simulink model "SAR_Quad_SITL_3D_v3"  (R2025b)
settings: Solver=ode4  StartTime=0.0  StopTime=inf  FixedStep=1/60  RelTol=1e-3
libraries: dspnetwork x5, sim3dlib x1, uavsim3dlib x1
(part 2 of 2)

== matlab function SAR_Quad_SITL_3D_v3/Edge_Command_Decoder ==
  data: raw_bytes input; target_pos_ned output size=3; gps_sensor_valid input; sim_time input; cur_pos input; cur_vel input; cur_eul input; cur_ang_vel input; min_lidar_range input; triage_code input; mission_phase output size=1; gps_valid_out output size=1; edge_ok output size=1; alt_nav_conf output size=1; yaw_cmd_deg output size=1; decoder_state output size=1; target_vel_ned output size=3; active_wp output size=1; planned_route_pts output size=[32 3]; num_route_pts output size=1
function [target_pos_ned, mission_phase, gps_valid_out, edge_ok, alt_nav_conf, yaw_cmd_deg, decoder_state, target_vel_ned, active_wp, planned_route_pts, num_route_pts] = Edge_Command_Decoder(raw_bytes, gps_sensor_valid, sim_time, cur_pos, cur_vel, cur_eul, cur_ang_vel, min_lidar_range, triage_code)
target_pos_ned = zeros(3, 1);
target_vel_ned = zeros(3, 1);
mission_phase  = 0.0;
gps_valid_out  = gps_sensor_valid;
edge_ok        = 1.0;
alt_nav_conf   = 0.95;
yaw_cmd_deg    = 0.0;
decoder_state  = 0.0;
active_wp      = 0.0;
planned_route_pts = zeros(32, 3);
num_route_pts  = 1.0;

persistent mode tgt_final user_yaw home_pos last_cmd_bytes is_init
persistent sp_pos sp_vel nav_phase
persistent corridor_wps num_corridor_wps corridor_idx smooth_yaw last_flight_yaw wp_stuck_timer
if isempty(is_init)
    is_init = true;
    mode = 0.0;
    tgt_final = [cur_pos(1); cur_pos(2); 0.0];
    user_yaw = cur_eul(3) * 180.0 / pi;
    smooth_yaw = cur_eul(3) * 180.0 / pi;
    last_flight_yaw = cur_eul(3) * 180.0 / pi;
    home_pos = [0.0; 0.0; -16.0];
    last_cmd_bytes = zeros(18, 1, 'uint8');
    sp_pos = [cur_pos(1); cur_pos(2); cur_pos(3)];
    sp_vel = [0.0; 0.0; 0.0];
    nav_phase = 0.0;
    corridor_wps = zeros(32, 3);
    corridor_wps(1, :) = [cur_pos(1), cur_pos(2), cur_pos(3)];
    num_corridor_wps = 1.0;
    corridor_idx = 1.0;
    wp_stuck_timer = 0.0;
end

% REALISTIC US CITY BLOCK GEOMETRY (Park quadrant [X: 115..190, Y: 10..90] open)
buildings = [
    -12.5,  46.0,   8.0,  80.0, -35.0, 0.0;   % Northwest Block 1
     54.0, 111.0,   8.0,  80.0, -35.0, 0.0;   % Northwest Block 2 (Red brick building)
    -12.5,  46.0, -80.0,  -8.0, -35.0, 0.0;   % Southwest Block 1
     54.0, 111.0, -80.0,  -8.0, -35.0, 0.0;   % Southwest Block 2
    195.0, 255.0,   8.0,  80.0, -35.0, 0.0;   % Far East Block (Perimeter boundary)
    129.0, 200.0, -80.0,  -8.0, -35.0, 0.0;   % Southeast Block
    -80.0, -29.0,   8.0,  80.0, -35.0, 0.0;   % West-North Block
    -80.0, -29.0, -80.0,  -8.0, -35.0, 0.0    % West-South Block
];

is_new = false;
if numel(raw_bytes) >= 18 && raw_bytes(1) == uint8(170)
    for k = 1:18
        if raw_bytes(k) ~= last_cmd_bytes(k)
            is_new = true; break;
        end
    end
else
    last_cmd_bytes = zeros(18, 1, 'uint8');
end

if is_new
    for k = 1:18; last_cmd_bytes(k) = raw_bytes(k); end
    cmd_id = double(raw_bytes(2));
    b1 = zeros(4, 1, 'uint8'); b2 = zeros(4, 1, 'uint8');
    b3 = zeros(4, 1, 'uint8'); b4 = zeros(4, 1, 'uint8');
    for bi = 1:4
        b1(bi) = raw_bytes(2 + bi); b2(bi) = raw_bytes(6 + bi);
        b3(bi) = raw_bytes(10 + bi); b4(bi) = raw_bytes(14 + bi);
    end
    p1 = double(typecast(b1, 'single'));
    p2 = double(typecast(b2, 'single'));
    p3 = double(typecast(b3, 'single'));
    p4 = double(typecast(b4, 'single'));

    plan_needed = false;
    search_needed = false;

    if cmd_id == 1.0 % TAKEOFF
        mode = 1.0;
        alt_target = max(2.5, abs(p3));
        tgt_final = [cur_pos(1); cur_pos(2); -alt_target];
        user_yaw = cur_eul(3) * 180.0 / pi;
        smooth_yaw = user_yaw;
        last_flight_yaw = user_yaw;
        nav_phase = 2.0;
        corridor_wps(1, :) = tgt_final';
        num_corridor_wps = 1.0;
        corridor_idx = 1.0;
    elseif cmd_id == 2.0 % HOLD
        mode = 2.0;
        tgt_final = [cur_pos(1); cur_pos(2); cur_pos(3)];
        user_yaw = cur_eul(3) * 180.0 / pi;
        nav_phase = 2.0;
    elseif cmd_id == 3.0 % GOTO
        mode = 3.0;
        tgt_final = [p1; p2; -abs(p3)];
        user_yaw = p4;
        plan_needed = true;
    elseif cmd_id == 4.0 % SEARCH
        mode = 4.0;
        tgt_final = [p1; p2; -abs(p3)];
        user_yaw = 0.0;
        search_needed = true;
    elseif cmd_id == 5.0 % RTL
        mode = 5.0;
        tgt_final = [home_pos(1); home_pos(2); home_pos(3)];
        user_yaw = 0.0;
        plan_needed = true;
    elseif cmd_id == 6.0 % LAND
        mode = 6.0;
        tgt_final = [cur_pos(1); cur_pos(2); 0.0];
        nav_phase = 2.0;
        corridor_wps(1, :) = tgt_final';
        num_corridor_wps = 1.0;
        corridor_idx = 1.0;
    end

    if search_needed
        z_search = tgt_final(3);
        cx = tgt_final(1); cy = tgt_final(2);
        corridor_wps = zeros(32, 3);
        corridor_wps(1, :) = [cur_pos(1), cur_pos(2), z_search];
        
        pat_type = p4;
        if pat_type >= 1.5
            % Creeping line sweep across the open park
            S = 12.0; L = 48.0;
            raw_wps = [
                cx - L/2, cy - S*2, z_search;
                cx + L/2, cy - S*2, z_search;
                cx + L/2, cy - S,   z_search;
                cx - L/2, cy - S,   z_search;
                cx - L/2, cy,       z_search;
                cx + L/2, cy,       z_search;
                cx + L/2, cy + S,   z_search;
                cx - L/2, cy + S,   z_search;
                cx - L/2, cy + S*2, z_search;
                cx + L/2, cy + S*2, z_search
            ];
        else
            S = 10.0;
            raw_wps = [
                cx,     cy,     z_search;
                cx + S, cy,     z_search;
                cx + S, cy + S, z_search;
                cx - S, cy + S, z_search;
                cx - S, cy - S, z_search;
                cx + 2*S, cy - S, z_search;
                cx + 2*S, cy + 2*S, z_search;
                cx - 2*S, cy + 2*S, z_search;
                cx - 2*S, cy - 2*S, z_search;
                cx + 3*S, cy - 2*S, z_search;
                cx + 3*S, cy + 3*S, z_search;
                cx - 3*S, cy + 3*S, z_search
            ];
        end
        
        nW = size(raw_wps, 1);
        SAFETY_MARGIN = 4.0;
        for wi = 1:nW
            wx = raw_wps(wi, 1); wy = raw_wps(wi, 2); wz = raw_wps(wi, 3);
            if wz > -34.0
                for bi = 1:size(buildings, 1)
                    bx1 = buildings(bi, 1) - SAFETY_MARGIN; bx2 = buildings(bi, 2) + SAFETY_MARGIN;
                    by1 = buildings(bi, 3) - SAFETY_MARGIN; by2 = buildings(bi, 4) + SAFETY_MARGIN;
                    if wx >= bx1 && wx <= bx2 && wy >= by1 && wy <= by2
                        d_faces = [abs(wx - bx1), abs(wx - bx2), abs(wy - by1), abs(wy - by2)];
                        [~, min_f] = min(d_faces);
                        if min_f == 1;     wx = bx1;
                        elseif min_f == 2; wx = bx2;
                        elseif min_f == 3; wy = by1;
                        else;              wy = by2;
                        end
                    end
                end
            end
            corridor_wps(wi + 1, :) = [wx, wy, wz];
        end
        num_corridor_wps = double(nW + 1);
        corridor_idx = 1.0;
        nav_phase = 1.0;
        wp_stuck_timer = 0.0;
    end

    if plan_needed
        z_target = tgt_final(3);
        c_x = cur_pos(1); c_y = cur_pos(2); c_z = cur_pos(3);
        t_x = tgt_final(1); t_y = tgt_final(2);
        
        direct_clear = false;
        if (z_target <= -34.0 && c_z <= -34.0)
            direct_clear = true;
        elseif (abs(c_y) <= 7.0 && abs(t_y) <= 7.0)
            direct_clear = true;
        elseif (abs(c_x - 120.0) <= 7.0 && abs(t_x - 120.0) <= 7.0)
            direct_clear = true;
        elseif (abs(c_x - 50.0) <= 3.5 && abs(t_x - 50.0) <= 3.5)
            direct_clear = true;
        elseif (abs(c_x + 20.0) <= 7.0 && abs(t_x + 20.0) <= 7.0)
            direct_clear = true;
        end
        
        if direct_clear
            corridor_wps = zeros(32, 3);
            corridor_wps(1, :) = [c_x, c_y, z_target];
            corridor_wps(2, :) = [t_x, t_y, z_target];
            num_corridor_wps = 2.0;
        else
            corr_axes = [-20.0, 50.0, 120.0];
            [~, idx_c] = min(abs(corr_axes - c_x));
            [~, idx_t] = min(abs(corr_axes - t_x));
            x_start_corr = corr_axes(idx_c);
            x_end_corr   = corr_axes(idx_t);
            
            corridor_wps = zeros(32, 3);
            corridor_wps(1, :) = [c_x, c_y, z_target];
            w_count = 1;
            if abs(c_y) > 6.0
                w_count = w_count + 1;
                corridor_wps(w_count, :) = [x_start_corr, c_y, z_target];
                w_count = w_count + 1;
                corridor_wps(w_count, :) = [x_start_corr, 0.0, z_target];
            else
                w_count = w_count + 1;
                corridor_wps(w_count, :) = [c_x, 0.0, z_target];
            end
            if abs(x_start_corr - x_end_corr) > 1.0
                w_count = w_count + 1;
                corridor_wps(w_count, :) = [x_end_corr, 0.0, z_target];
            end
            if abs(t_y) > 6.0
                w_count = w_count + 1;
                corridor_wps(w_count, :) = [x_end_corr, t_y, z_target];
            end
            w_count = w_count + 1;
            corridor_wps(w_count, :) = [t_x, t_y, z_target];
            num_corridor_wps = double(w_count);
        end
        corridor_idx = 1.0;
        nav_phase = 1.0;
        wp_stuck_timer = 0.0;
    end
end

if mode < 0.5
    target_pos_ned = [cur_pos(1); cur_pos(2); cur_pos(3)];
    target_vel_ned = [0.0; 0.0; 0.0];
    sp_pos = [cur_pos(1); cur_pos(2); cur_pos(3)];
    sp_vel = [0.0; 0.0; 0.0];
    yaw_cmd_deg = user_yaw;
    mission_phase = 0.0;
    active_wp = 0.0;
    decoder_state = 0.0;
    planned_route_pts = corridor_wps;
    num_route_pts = num_corridor_wps;
    return;
end

c_idx = int32(corridor_idx);
if c_idx < 1; c_idx = int32(1); end
if c_idx > int32(num_corridor_wps); c_idx = int32(num_corridor_wps); end
active_target_pos = corridor_wps(c_idx, :)';

dist_wp_actual = norm(active_target_pos(1:2) - cur_pos(1:2));
dist_wp_sp     = norm(active_target_pos(1:2) - sp_pos(1:2));
cur_speed_xy   = norm(cur_vel(1:2));
dt = 1/60;

% UNREACHABLE WAYPOINT TIMEOUT: Advance if progress stalls near a wall
if c_idx < int32(num_corridor_wps)
    if dist_wp_actual > 2.0 && min_lidar_range < 3.5 && cur_speed_xy < 0.50
        wp_stuck_timer = wp_stuck_timer + dt;
    else
        wp_stuck_timer = max(0.0, wp_stuck_timer - 0.5 * dt);
    end
    if wp_stuck_timer > 0.90
        c_idx = c_idx + 1;
        corridor_idx = double(c_idx);
        active_target_pos = corridor_wps(c_idx, :)';
        wp_stuck_timer = 0.0;
    end
end

corner_angle_deg = 0.0;
if c_idx < int32(num_corridor_wps)
    next_wp = corridor_wps(c_idx + 1, :)';
    v_in = active_target_pos(1:2) - sp_pos(1:2);
    v_out = next_wp(1:2) - active_target_pos(1:2);
    if norm(v_in) > 0.1 && norm(v_out) > 0.1
        cos_ang = dot(v_in, v_out) / (norm(v_in) * norm(v_out));
        cos_ang = max(-1.0, min(1.0, cos_ang));
        corner_angle_deg = acos(cos_ang) * 180.0 / pi;
    end
end

r_switch = max(2.0, min(4.2, 0.28 * cur_speed_xy));
if c_idx < int32(num_corridor_wps)
    if (dist_wp_actual < r_switch && dist_wp_sp < r_switch * 1.2)
        c_idx = c_idx + 1;
        corridor_idx = double(c_idx);
        active_target_pos = corridor_wps(c_idx, :)';
        wp_stuck_timer = 0.0;
    end
end

speed_xy = norm(sp_vel(1:2));
if abs(user_yaw) > 1e-3
    desired_yaw = user_yaw;
    last_flight_yaw = user_yaw;
elseif speed_xy > 0.50
    desired_yaw = atan2(sp_vel(2), sp_vel(1)) * 180.0 / pi;
    last_flight_yaw = desired_yaw;
else
    desired_yaw = last_flight_yaw;
end
dyaw = atan2(sin((desired_yaw - smooth_yaw)*pi/180), cos((desired_yaw - smooth_yaw)*pi/180)) * 180 / pi;
MAX_YAW_RATE = 180.0;
max_dyaw_step = MAX_YAW_RATE * dt;
if abs(dyaw) > max_dyaw_step
    smooth_yaw = smooth_yaw + sign(dyaw) * max_dyaw_step;
else
    smooth_yaw = desired_yaw;
end

% =========================================================================
% DYNAMIC SMART SPEED GOVERNOR (Distance & Task Adaptive)
% =========================================================================
d_goal_total = norm(active_target_pos(1:2) - cur_pos(1:2));

% Tier 1: Task and Distance Urgency
if triage_code == 1.0 % PRIORITY RED SOS DIVERSION
    v_task_max = 18.0; % Emergency sprint
elseif mode == 3.0 || mode == 5.0 % TRANSIT GOTO OR RTL
    if d_goal_total > 35.0
        v_task_max = 17.5; % Long-haul transit sprint
    elseif d_goal_total > 15.0
        v_task_max = 12.0;
    else
        v_task_max = 7.0;
    end
elseif mode == 4.0 % ACTIVE SAR SWEEP
    v_task_max = 8.5;  % Search speed for optimal camera exposure
else
    v_task_max = 6.0;
end

% Tier 2: LiDAR Obstacle Clearance De-Rating
d_safe = max(0.5, min_lidar_range - 2.0);
v_obs_safe = sqrt(2.0 * 2.8 * d_safe);

% Tier 3: Tilt-Bounded Corner Entry Deceleration (Clamps tilt <= 20 deg)
if corner_angle_deg > 25.0
    v_corner_limit = max(3.5, v_task_max * cos(corner_angle_deg * pi / 360.0));
    v_entry_max = sqrt(v_corner_limit^2 + 2.0 * 2.8 * dist_wp_sp);
else
    v_entry_max = v_task_max;
end

V_MAX_XY = min([v_task_max, v_obs_safe, v_entry_max]);
A_MAX_XY = 3.5; % Matched acceleration for 20 deg tilt (g * tan(20 deg) = 3.57 m/s^2)
V_MAX_DN = 3.0; V_MAX_UP = 4.5;
A_MAX_DN = 2.5; A_MAX_UP = 3.5;

delta_xy = active_target_pos(1:2) - sp_pos(1:2);
dist_xy  = norm(delta_xy);
if dist_xy > 0.02
    dir_xy = delta_xy / dist_xy;
    v_des_mag_xy = min(V_MAX_XY, sqrt(2.0 * A_MAX_XY * dist_xy));
    v_des_xy = dir_xy * v_des_mag_xy;
else
    v_des_xy = [0.0; 0.0];
end
dv_xy = v_des_xy - sp_vel(1:2);
dv_mag_xy = norm(dv_xy);
max_step_dv_xy = A_MAX_XY * dt;
if dv_mag_xy > max_step_dv_xy
    sp_vel(1:2) = sp_vel(1:2) + (dv_xy / dv_mag_xy) * max_step_dv_xy;
else
    sp_vel(1:2) = v_des_xy;
end
sp_pos(1:2) = sp_pos(1:2) + sp_vel(1:2) * dt;

leash_err = sp_pos(1:2) - cur_pos(1:2);
leash_dist = norm(leash_err);
MAX_LEASH = 3.5;
if leash_dist > MAX_LEASH
    sp_pos(1:2) = cur_pos(1:2) + (leash_err / leash_dist) * MAX_LEASH;
    sp_vel(1:2) = sp_vel(1:2) * (MAX_LEASH / leash_dist);
end

delta_z = active_target_pos(3) - sp_pos(3);
if delta_z > 0.0
    v_des_z = min(V_MAX_DN, sqrt(2.0 * A_MAX_DN * delta_z));
    a_limit_z = A_MAX_DN;
else
    v_des_z = -min(V_MAX_UP, sqrt(2.0 * A_MAX_UP * (-delta_z)));
    a_limit_z = A_MAX_UP;
end
dv_z = v_des_z - sp_vel(3);
max_step_dv_z = a_limit_z * dt;
if abs(dv_z) > max_step_dv_z
    sp_vel(3) = sp_vel(3) + sign(dv_z) * max_step_dv_z;
else
    sp_vel(3) = v_des_z;
end
sp_pos(3) = sp_pos(3) + sp_vel(3) * dt;

target_pos_ned = [sp_pos(1); sp_pos(2); sp_pos(3)];
target_vel_ned = [sp_vel(1); sp_vel(2); sp_vel(3)];
yaw_cmd_deg    = smooth_yaw;
mission_phase  = mode;
active_wp      = corridor_idx;
decoder_state  = nav_phase;
planned_route_pts = corridor_wps;
num_route_pts  = num_corridor_wps;

== stateflow chart SAR_Quad_SITL_3D_v3/Supervisor_Stateflow ==
  state GPS_PRIMARY
    entry: nav_mode = 0;
  state VIO_TERCOM_NAV
    entry: nav_mode = 1;
  state INERTIAL_HOLD
    entry: nav_mode = 2;
  (default) -> GPS_PRIMARY
  INERTIAL_HOLD -> GPS_PRIMARY : [gps_valid >= 0.5]
  VIO_TERCOM_NAV -> GPS_PRIMARY [order 1] : [gps_valid >= 0.5]
  GPS_PRIMARY -> VIO_TERCOM_NAV [order 1] : [gps_valid < 0.5 && alt_nav_conf >= 0.55]
  GPS_PRIMARY -> INERTIAL_HOLD [order 2] : [gps_valid < 0.5 && alt_nav_conf < 0.55]
  VIO_TERCOM_NAV -> INERTIAL_HOLD [order 2] : [alt_nav_conf < 0.55]
  data: gps_valid input double; alt_nav_conf input double; nav_mode output double

== matlab function SAR_Quad_SITL_3D_v3/TERCOM_Nav_System ==
  data: cur_pos input; est_pos output size=3; cur_vel input; cur_eul input; gps_valid input; sim_time input; vo_vel input; vo_conf input; est_vel output size=3; alt_nav_conf output size=1; tercom_fix_pos output size=3; h_agl output size=1; dem_elev output size=1; nav_mode_status output size=1
function [est_pos, est_vel, alt_nav_conf, tercom_fix_pos, h_agl, dem_elev, nav_mode_status] = TERCOM_Nav_System(cur_pos, cur_vel, cur_eul, gps_valid, sim_time, vo_vel, vo_conf)
est_pos = [0.0; 0.0; 0.0]; est_vel = [0.0; 0.0; 0.0];
alt_nav_conf = 0.95; tercom_fix_pos = [0.0; 0.0; 0.0];
h_agl = 0.0; dem_elev = 0.0; nav_mode_status = 0.0;
persistent p_nom v_nom R_nom ba_nom bg_nom P_cov
persistent last_time last_vel_truth fix_pos
if isempty(P_cov)
    p_nom = [0; 0; 0]; v_nom = [0; 0; 0]; R_nom = eye(3);
    ba_nom = [0.06; -0.05; 0.02]; bg_nom = [0.004; -0.003; 0.002];
    P_cov = blkdiag(0.15*eye(3), 0.04*eye(3), 0.01*eye(3), 0.05*eye(3), 0.001*eye(3));
    last_time = sim_time; last_vel_truth = cur_vel; fix_pos = cur_pos;
end
dt = sim_time - last_time;
if dt <= 0.0 || dt > 0.1; dt = 1/60; end
last_time = sim_time;

dem_elev = 2.4 * sin(0.035 * cur_pos(1)) * cos(0.035 * cur_pos(2)) + 1.2 * sin(0.07 * cur_pos(1));
true_agl = max(0.0, -cur_pos(3) - dem_elev);
h_agl = true_agl + 0.03 * sin(sim_time * 12.0);

a_truth = (cur_vel - last_vel_truth) / dt;
last_vel_truth = cur_vel;
f_spec_world = a_truth - [0; 0; 9.81];
phi = cur_eul(1); theta = cur_eul(2); psi = cur_eul(3);
R_truth = [cos(theta)*cos(psi), sin(phi)*sin(theta)*cos(psi)-cos(phi)*sin(psi), cos(phi)*sin(theta)*cos(psi)+sin(phi)*sin(psi);
           cos(theta)*sin(psi), sin(phi)*sin(theta)*sin(psi)+cos(phi)*cos(psi), cos(phi)*sin(theta)*sin(psi)-sin(phi)*cos(psi);
          -sin(theta),          sin(phi)*cos(theta),                            cos(phi)*cos(theta)];
f_b_meas = R_truth' * f_spec_world + ba_nom + 0.02 * [sin(sim_time*30); cos(sim_time*25); sin(sim_time*20)];
w_b_meas = [0; 0; 0] + bg_nom + 0.001 * [cos(sim_time*15); sin(sim_time*15); cos(sim_time*10)];

f_b_corr = f_b_meas - ba_nom; w_b_corr = w_b_meas - bg_nom;
w_skew = [0, -w_b_corr(3), w_b_corr(2); w_b_corr(3), 0, -w_b_corr(1); -w_b_corr(2), w_b_corr(1), 0];
R_nom = R_nom * (eye(3) + w_skew * dt);
a_nom_world = R_nom * f_b_corr + [0; 0; 9.81];
p_nom = p_nom + v_nom * dt + 0.5 * a_nom_world * (dt^2);
v_nom = v_nom + a_nom_world * dt;
if p_nom(3) > 0.0; p_nom(3) = 0.0; v_nom(3) = 0.0; end

f_skew = [0, -f_b_corr(3), f_b_corr(2); f_b_corr(3), 0, -f_b_corr(1); -f_b_corr(2), f_b_corr(1), 0];
F = eye(15); F(1:3, 4:6) = eye(3)*dt; F(4:6, 7:9) = -R_nom*f_skew*dt; F(4:6, 10:12) = -R_nom*dt; F(7:9, 7:9) = eye(3)-w_skew*dt; F(7:9, 13:15) = -eye(3)*dt;
Q = blkdiag(1e-4*eye(3), 0.02*eye(3), 1e-4*eye(3), 1e-5*eye(3), 1e-6*eye(3)) * dt;
P_cov = F * P_cov * F' + Q;

if gps_valid >= 0.5
    z_gps = [cur_pos; cur_vel]; H_gps = [eye(6), zeros(6, 9)]; R_gps = blkdiag(0.18*eye(3), 0.04*eye(3));
    y_gps = z_gps - [p_nom; v_nom]; S_gps = H_gps * P_cov * H_gps' + R_gps; K_gps = P_cov * H_gps' / S_gps;
    dx_gps = K_gps * y_gps;
    p_nom = p_nom + dx_gps(1:3); v_nom = v_nom + dx_gps(4:6);
    dth = dx_gps(7:9); dth_skew = [0, -dth(3), dth(2); dth(3), 0, -dth(1); -dth(2), dth(1), 0];
    R_nom = R_nom * (eye(3) + dth_skew);
    ba_nom = ba_nom + dx_gps(10:12); bg_nom = bg_nom + dx_gps(13:15);
    P_cov = (eye(15) - K_gps * H_gps) * P_cov;
    fix_pos = p_nom; nav_mode_status = 0.0;
else
    if vo_conf >= 0.30
        H_vo = [zeros(3,3), eye(3), zeros(3,9)]; R_vo = diag([0.06, 0.06, 0.10]) / max(vo_conf, 0.1);
        y_vo = vo_vel - v_nom; S_vo = H_vo * P_cov * H_vo' + R_vo; K_vo = P_cov * H_vo' / S_vo;
        dx_vo = K_vo * y_vo;
        p_nom = p_nom + dx_vo(1:3); v_nom = v_nom + dx_vo(4:6);
        P_cov = (eye(15) - K_vo * H_vo) * P_cov;
    end
    fix_pos = p_nom; nav_mode_status = 1.0;
end

cov_trace_pos = trace(P_cov(1:3, 1:3));
alt_nav_conf = max(0.15, min(0.98, exp(-0.045 * cov_trace_pos)));
tercom_fix_pos = fix_pos; est_pos = p_nom; est_vel = v_nom;
